simulink model "CommsModel"  (R2019b)
settings: Solver=VariableStepAuto  StartTime=0.0  StopTime=2.1e-07  RelTol=1e-3
model workspace (MAT data in the model file):
  PiFc = 6283.18530718
values from neighbouring files (symbols this model uses):
  Fc = 2.4e9    (= 2400000000)    [main.m]
  SampSin = Tb/wperiod    (= 8.33333333333e-12)    [main.m]
  tau = 1/(2*pi*(Fc+1e9))    (= 4.681027738e-11)    [main.m]
  Tb = 1/(Fc)    (= 4.16666666667e-10)    [main.m]
  wperiod = 50    [main.m]
libraries: dspsigops x2, simulink x1, commfilt2 x1, simulink_extras x1, commsink2 x1, commrflib2 x1
settings Model: Creator=pranaviboyalakuntla  LastModifiedBy=pranaviboyalakuntla
settings DataIOCC: ExternalInput=bits  LoadExternalInput=on

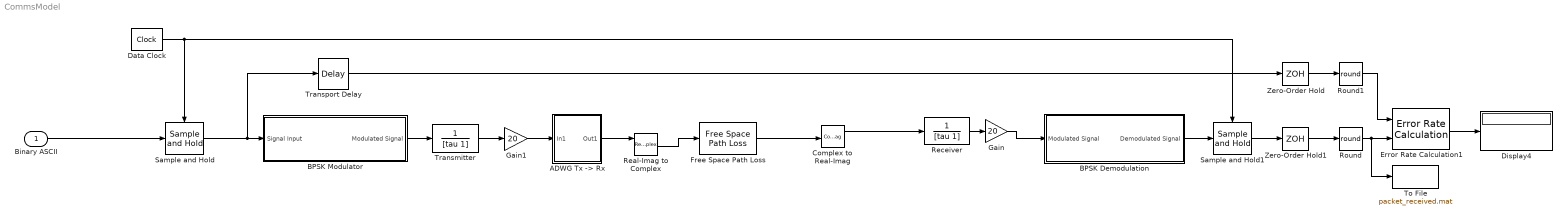
== system CommsModel ==
  Binary ASCII : Inport  Interpolate=off
  "ADWG Tx -> Rx" : Subsystem
  "BPSK Demodulation " : Subsystem
  BPSK Modulator : Subsystem
  Complex to Real-Imag : ComplexToRealImag
  Data Clock : simulink_extras/Flip Flops/Clock  period=Tb
  Display4 : Display
  Error Rate Calculation1 : commsink2/Error Rate Calculation  N=0  st_delay=0  cp_mode=Entire frame  subframe=[]  PMode=Port  WsName=ErrorVec  RsMode2=off  stop=off  numErr=100  maxBits=1e6
      settings: SourceProductName=Communications Toolbox
  Free Space Path Loss : commrflib2/Free Space Path Loss  mode=Decibels  dB=60  d=0.01  fc=loss
      settings: SourceProductName=Communications Toolbox  SourceProductBaseCode=CM
  Gain : Gain  Gain=20
  Gain1 : Gain  Gain=20
  Real-Imag to Complex : RealImagToComplex
  Receiver : TransferFcn  Denominator=[tau 1]
  Round : Rounding  Operator=round
  Round1 : Rounding  Operator=round
  Sample and Hold : dspsigops/Sample and Hold  trig=Rising edge  initCond=0  latchinput=on
  Sample and Hold1 : dspsigops/Sample and Hold  trig=Rising edge  initCond=0  latchinput=on
  To File : ToFile  Filename=packet_received.mat  MatrixName=packet_received
  Transmitter : TransferFcn  Denominator=[tau 1]
  Transport Delay : TransportDelay  DelayTime=Tb
  Zero-Order Hold : ZeroOrderHold  SampleTime=Tb
  Zero-Order Hold1 : ZeroOrderHold  SampleTime=Tb
  wires:
  Data Clock/1 -> Sample and Hold/Trigger, Sample and Hold1/Trigger
  Binary ASCII/1 -> Sample and Hold/1
  Zero-Order Hold1/1 -> Round/1
  Round/1 -> To File/1, Error Rate Calculation1/2
  Error Rate Calculation1/1 -> Display4/1
  "BPSK Demodulation "/1(Demodulated Signal) -> Sample and Hold1/1
  Sample and Hold1/1 -> Zero-Order Hold1/1
  Zero-Order Hold/1 -> Round1/1
  Round1/1 -> Error Rate Calculation1/1
  Sample and Hold/1 -> Transport Delay/1, BPSK Modulator/1(Signal Input)
  Transport Delay/1 -> Zero-Order Hold/1
  BPSK Modulator/1(Modulated Signal) -> Transmitter/1
  Transmitter/1 -> Gain1/1
  Receiver/1 -> Gain/1
  "ADWG Tx -> Rx"/1(Out1) -> Real-Imag to Complex/1
  Real-Imag to Complex/1 -> Free Space Path Loss/1
  Free Space Path Loss/1 -> Complex to Real-Imag/1
  Complex to Real-Imag/1 -> Receiver/1
  Gain/1 -> "BPSK Demodulation "/1("Modulated Signal ")
  Gain1/1 -> "ADWG Tx -> Rx"/1(In1)

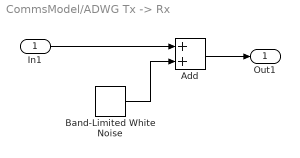
== system CommsModel/ADWG Tx -> Rx ==
  In1 : Inport
  Add : Sum
  Band-Limited White Noise : simulink/Sources/Band-Limited White Noise  Cov=[2e-20]  Ts=SampSin  seed=[0.3]
  Out1 : Outport
  wires:
  Add/1 -> Out1/1
  In1/1 -> Add/1
  Band-Limited White Noise/1 -> Add/2

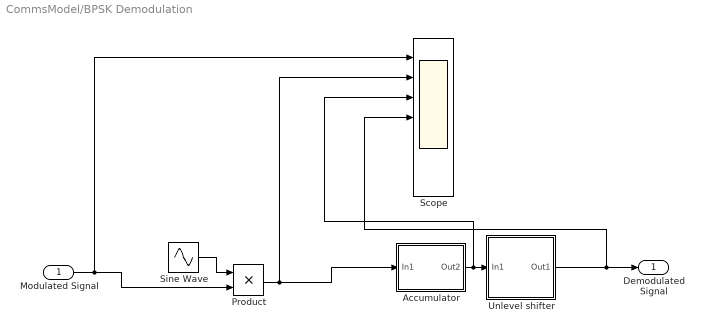
== system CommsModel/BPSK Demodulation  ==
  "Modulated Signal " : Inport
  Accumulator : Subsystem
  Product : Product
  Scope : Scope  NumInputPorts=7
  Sine Wave : Sin  Frequency=Fc * 2 * pi  Phase=pi  SampleTime=SampSin
  "Unlevel shifter " : Subsystem
  Demodulated Signal : Outport
  wires:
  Sine Wave/1 -> Product/1
  "Modulated Signal "/1 -> Scope/1, Product/2
  Product/1 -> Scope/2, Accumulator/1(In1)
  Accumulator/1(Out2) -> Scope/3, "Unlevel shifter "/1(In1)
  "Unlevel shifter "/1(Out1) -> Scope/4, Demodulated Signal/1

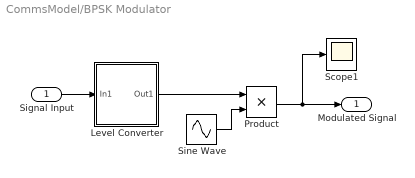
== system CommsModel/BPSK Modulator ==
  Signal Input : Inport
  Level Converter : Subsystem
  Product : Product
  Scope1 : Scope
  Sine Wave : Sin  Frequency=Fc * 2 * pi  Phase=pi  SampleTime=SampSin
  Modulated Signal : Outport
  wires:
  Sine Wave/1 -> Product/2
  Product/1 -> Scope1/1, Modulated Signal/1
  Signal Input/1 -> Level Converter/1(In1)
  Level Converter/1(Out1) -> Product/1

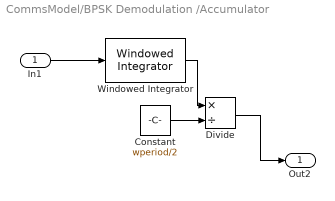
== system CommsModel/BPSK Demodulation /Accumulator ==
  In1 : Inport
  Constant : Constant  Value=wperiod/2
  Divide : Product  Inputs=*/
  Windowed Integrator : commfilt2/Windowed Integrator  integperiod=wperiod  InputProcessing=Columns as channels (frame based)  roundingMode=Floor  overflowMode=off  coeffDataTypeStr=Inherit: Same word length as input  coeffMin=[]  coeffMax=[]  coeffLastDataTypeStr=Inherit: Same word length as input  accumDataTypeStr=Inherit: Same as product output  accumLastDataTypeStr=Inherit: Same as product output  outputDataTypeStr=Inherit: Same as accumulator  outputMin=[]  outputMax=[]  outputLastDataTypeStr=Inherit: Same as accumulator
      settings: SourceProductName=Communications Toolbox  SourceProductBaseCode=CM
  Out2 : Outport
  wires:
  Divide/1 -> Out2/1
  Constant/1 -> Divide/2
  In1/1 -> Windowed Integrator/1
  Windowed Integrator/1 -> Divide/1

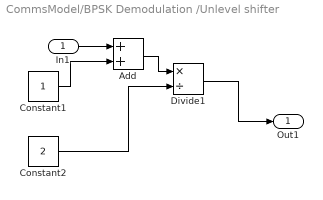
== system CommsModel/BPSK Demodulation /Unlevel shifter  ==
  In1 : Inport
  Add : Sum
  Constant1 : Constant
  Constant2 : Constant  Value=2
  Divide1 : Product  Inputs=*/
  Out1 : Outport
  wires:
  Divide1/1 -> Out1/1
  In1/1 -> Add/1
  Constant1/1 -> Add/2
  Constant2/1 -> Divide1/2
  Add/1 -> Divide1/1

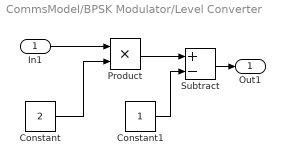
== system CommsModel/BPSK Modulator/Level Converter ==
  In1 : Inport
  Constant : Constant  Value=2
  Constant1 : Constant
  Product : Product
  Subtract : Sum  Inputs=+-
  Out1 : Outport
  wires:
  Constant/1 -> Product/2
  Constant1/1 -> Subtract/2
  Subtract/1 -> Out1/1
  In1/1 -> Product/1
  Product/1 -> Subtract/1
